simulink model "AndyVodynsyssim"  (R2021b)
settings: Solver=FixedStepAuto  StartTime=0.0  StopTime=20  RelTol=1e-3
settings Model: Creator=andyvo  LastModifiedBy=andyvo

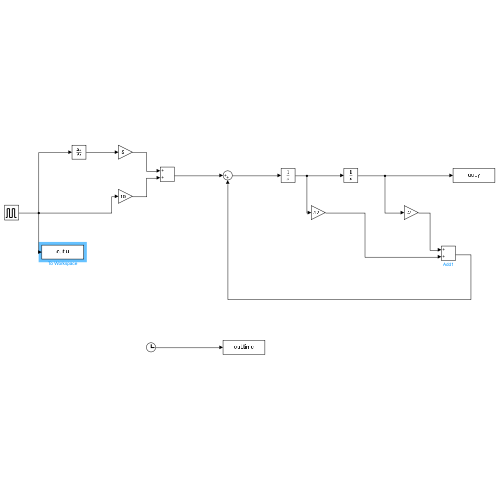
[thumbnail: Simulink's stored preview of the top-level diagram]
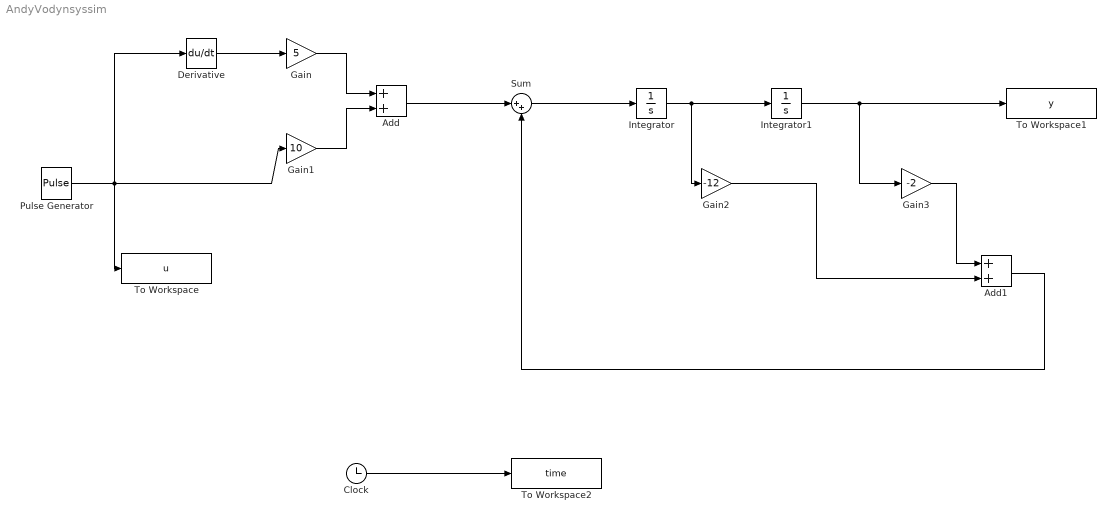
== system AndyVodynsyssim ==
  Add : Sum
  Add1 : Sum
  Clock : Clock
      settings: Decimation=30
  Derivative : Derivative  CoefficientInTFapproximation=10
  Gain : Gain  Gain=5
  Gain1 : Gain  Gain=10
  Gain2 : Gain  Gain=-12
  Gain3 : Gain  Gain=-2
  Integrator : Integrator
  Integrator1 : Integrator
  Pulse Generator : DiscretePulseGenerator  PulseType=Time based  Amplitude=10  Period=20  PulseWidth=50
  Sum : Sum  Inputs=|++
  To Workspace : ToWorkspace  VariableName=u  SampleTime=-1
  To Workspace1 : ToWorkspace  VariableName=y  SampleTime=-1
  To Workspace2 : ToWorkspace  VariableName=time  SampleTime=-1
  wires:
  Derivative/1 -> Gain/1
  Gain/1 -> Add/1
  Gain1/1 -> Add/2
  Pulse Generator/1 -> Derivative/1, Gain1/1, To Workspace/1
  Add/1 -> Sum/1
  Gain3/1 -> Add1/1
  Gain2/1 -> Add1/2
  Add1/1 -> Sum/2
  Sum/1 -> Integrator/1
  Integrator/1 -> Gain2/1, Integrator1/1
  Integrator1/1 -> To Workspace1/1, Gain3/1
  Clock/1 -> To Workspace2/1
